simulink model "Reaching"  (R2024b)
settings: Solver=FixedStepDiscrete  StartTime=0.0  StopTime=inf  FixedStep=0.001  RelTol=1e-3
undefined symbols (not defined in the file): get
libraries: PhanTorque_3Dof_Library_64Bits x1, vrlib x1
settings Model: Creator=carlos.aldana  LastModifiedBy=philg
settings SolverCC: AlgebraicLoopSolver=TrustRegion
settings DataIOCC: LimitDataPoints=on  SaveFormat=Array  ReturnWorkspaceOutputs=off
settings OptimizationCC: BlockReduction=off  BooleanDataType=off  LifeSpan=inf
settings DebuggingCC: SaveWithParameterizedLinksMsg=none  UnderspecifiedInitializationDetection=Classic  MergeDetectMultiDrivingBlocksExec=none  SignalResolutionControl=TryResolveAllWithWarning  UnconnectedInputMsg=warning  UnconnectedOutputMsg=warning  UnconnectedLineMsg=warning  AllowSymbolicDim=off  SFUnexpectedBacktrackingDiag=warning  SFNoUnconditionalDefaultTransitionDiag=warning  SFExecutionAtInitializationDiag=none  ArithmeticOperatorsInVariantConditions=warning
settings HardwareCC: ProdBitPerPointer=32  ProdBitPerSizeT=32  ProdBitPerPtrDiffT=32  ProdLargestAtomicFloat=None  ProdIntDivRoundTo=Undefined  ProdEndianess=Unspecified  ProdWordSize=32  ProdHWDeviceType=32-bit Generic  TargetUnknown=on
settings ModelReferenceCC: EnableRefExpFcnMdlSchedulingChecks=on  PropagateSignalLabelsOutOfModel=off
settings SFSimCC: SimUseLocalCustomCode=off  CustomCodeUndefinedFunction=UseInterfaceOnly
settings RTWCC: RTWUseLocalCustomCode=off  GPUComputeCapability=3.5  DLArmComputeVersion=19.05
settings CodeAppCC: StateflowObjectComments=on
settings GRTTargetCC: TargetLangStandard=C89/C90 (ANSI)
settings ConfigComp: CovMetricSettings=dw  CovSaveCumulativeToWorkspaceVar=on  CovSaveSingleToWorkspaceVar=on  CovExternalEMLEnable=off  CovSFcnEnable=off

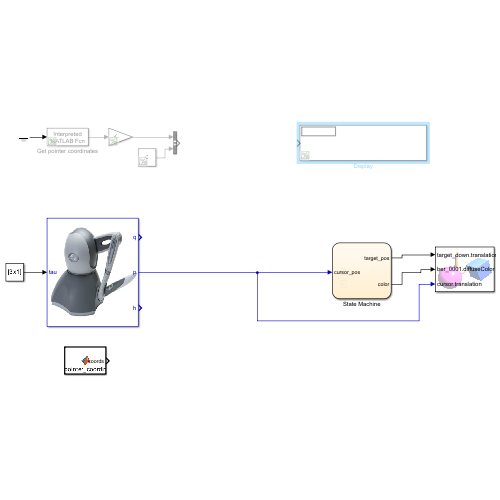
[thumbnail: Simulink's stored preview of the top-level diagram]
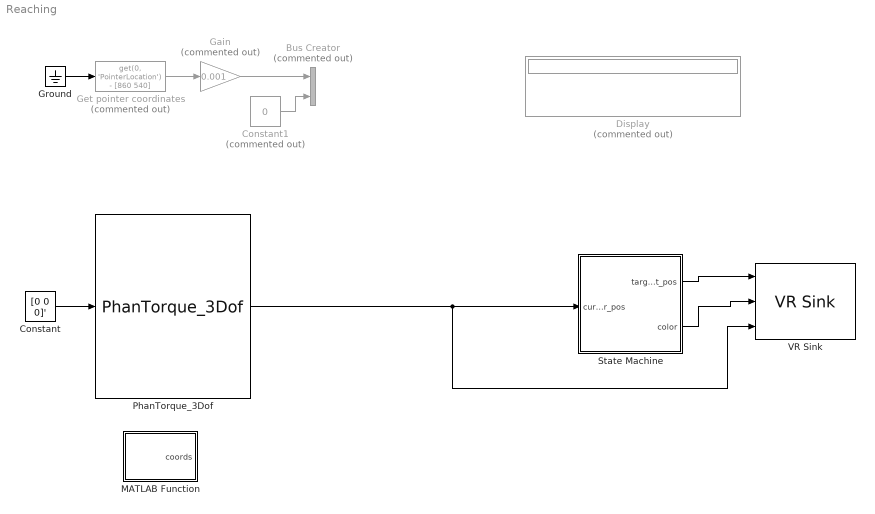
== system Reaching ==
  Bus Creator : BusCreator  Commented=on  Inputs=2
  Constant : Constant  Value=[0 0 0]'
  Constant1 : Constant  Commented=on  Value=0
  Display : Display  Commented=on
  Gain : Gain  Commented=on  Gain=0.001
  Get pointer coordinates : MATLABFcn  Commented=on  MATLABFcn=get(0, 'PointerLocation') - [860 540]  OutputDimensions=2
  Ground : Ground
  MATLAB Function : MATLAB Function  TreatAsAtomicUnit=on
  PhanTorque_3Dof : PhanTorque_3Dof_Library_64Bits/PhanTorque_3Dof  Haptic_Name='Default Device'
  State Machine : Stateflow chart  TreatAsAtomicUnit=on
  VR Sink : vrlib/VR Sink  InstantiateOnLoad=on  SampleTime=0.1  ViewEnable=on  RemoteChange=off  RemoteView=off  FieldsWritten=target_down.translation.3.1.1.double#ber_0001.diffuseColor.3.1.1.double#cursor.translation.3.1.1.double  WorldFileName=VR_centerAndTarget.wrl  AutoView=off  VideoDimensions=[]  AllowVariableSize=off
  wires:
  Get pointer coordinates/1 -> Gain/1
  Ground/1 -> Get pointer coordinates/1
  State Machine/1(target_pos) -> VR Sink/1
  State Machine/2(color) -> VR Sink/2
  Constant/1 -> PhanTorque_3Dof/1
  Gain/1 -> Bus Creator/1
  Constant1/1 -> Bus Creator/2
  PhanTorque_3Dof/2 -> VR Sink/3, State Machine/1(cursor_pos)

== stateflow chart Reaching/State Machine ==
  state Initializing [commented out]
    entry:
    counter = 0;
    time = 0;
    color = [0 1 1];
    radius = 0.1;
  state HOME2 [commented out]
    target_pos=[0,0,0]';
    target_color=[1 0 0];
  state WAIT_HOME1 [commented out]
  state REACHING2 [commented out]
    % Calcola un target random sul cerchio di raggio 0.1m (10cm)
    theta = rand() * 2 * pi;
    target_pos = [0.1 * cos(theta); 0.1 * sin(theta); 0];
  state INIT
    entry:
    counter = 0;
    radius = 0.1;
    target_pos = [0 0 0];
    color = [1 0 0]; % Rosso
  state FEEDBACK2 [commented out]
    target_color = [0 1 0];  % Diventa Verde
  state New_target [commented out]
    entry:
  state Finish1 [commented out]
  state GO_HOME
    entry:
    target_pos = [0 0 0];
    color = [1 0 0]; % Rosso
  state HOLD_HOME
    color = [0 1 0]; % Verde (Holding)
  state CALC_NEW_TARGET
    % Calcola l'angolo: 0, 45, 90...
    entry:
    theta = randi(8) * (pi/4);
    target_pos(1) = radius * cos(theta);
    target_pos(2) = radius * sin(theta);
    target_pos(3) = 0;
    color = [1 0 1]; % Magenta target attivo)
  state REACHING
    entry:
    color = [1 0 1]; % Forza Magenta
  state HOLD_TARGET
    entry:
    color = [0 1 0]; % Verde (Preso!)
  state FINISH
    entry:
    target_pos = [0 0 0];
    color = [0 0 1]; % Blu (Finito tutto)
  (default) -> Initializing [commented out]
  Initializing -> HOME2 [commented out]
  FEEDBACK2 -> HOME2 [commented out] : [after(1,sec)]{counter = counter + 1}
  HOME2 -> WAIT_HOME1 [commented out] : [norm(cursor_pos-target_pos) < 0.005]
  WAIT_HOME1 -> REACHING2 [commented out] : [after(1,sec)]
  REACHING2 -> FEEDBACK2 [commented out] : [norm(cursor_pos - target_pos) < 0.005]
  (default) -> INIT
  FEEDBACK2 -> Finish1 [commented out] : [counter >= 10]
  INIT -> GO_HOME
  (junction 43) -> GO_HOME [order 2]
  GO_HOME -> HOLD_HOME : [sqrt((cursor_pos(1)-target_pos(1))^2 + (cursor_pos(2)-target_pos(2))^2) < 0.02]
  HOLD_HOME -> CALC_NEW_TARGET : after(2,sec)
  CALC_NEW_TARGET -> REACHING
  REACHING -> HOLD_TARGET : [[sqrt((cursor_pos(1)-target_pos(1))^2 + (cursor_pos(2)-target_pos(2))^2) < 0.02]]
  HOLD_TARGET -> (junction 43) : [after(1, sec)]{counter = counter + 1;}
  (junction 43) -> FINISH [order 1] : [counter >= 8]
  data: data local; radius local; theta local; target_pos output; target_color local; counter local; angle local; color output =[1 0 0]; time local; cursor_pos input size=[3 1]

== matlab function Reaching/MATLAB Function ==
  data: coords output
% function coords = get_pointer_coordinates
%     coords = get(0, 'PointerLocation'); 



function coords = get_pointer_coordinates
    % Diciamo a Simulink che 'get' è una funzione esterna
    coder.extrinsic('get');
    
    % Dobbiamo inizializzare la variabile (altrimenti Simulink non sa quanto è grande)
    temp = zeros(1, 2); 
    
    % Leggiamo il mouse
    temp = get(0, 'PointerLocation');
    
    % Aggiungiamo uno zero per la Z (perché il robot vuole X, Y, Z)
    % e trasponiamo con l'apice ' per avere un vettore colonna
    coords = [temp, 0]'; 
end
